simulink model "MMC_SimpleModel_20250505"  (R2024b)
settings: Solver=VariableStepAuto  StartTime=0.0  StopTime=0.5  RelTol=1e-3
values from neighbouring files (symbols this model uses):
  a = 1    [param_allsim_20250429.m]
  f0 = 50    [param_allsim_20250429.m]
  L_ac = 100e-6    (= 0.0001)    [param_allsim_20250429.m]
  L_arm = 1e-3    (= 0.001)    [param_allsim_20250429.m]
  m = 1    [param_allsim_20250429.m]
  R = 1e-6    (= 1e-06)    [param_allsim_20250429.m]
  R_ac = 1    [param_allsim_20250429.m]
  R_arm = 1e-2    (= 0.01)    [param_allsim_20250429.m]
  VDC = 800    [param_allsim_20250429.m]
undefined symbols (not defined in the file or in its folder): C_SM, L
libraries: spsSeriesRLCBranchLib x8, spsCurrentMeasurementLib x7, spsControlledVoltageSourceLib x6, spsVoltageMeasurementLib x4, spsDCVoltageSourceLib x2, spsGroundLib x1, spsThreePhaseSeriesRLCBranchLib x1, spsThreePhaseVIMeasurementLib x1, spspowerguiLib x1
settings Model: Creator=ana  LastModifiedBy=ana

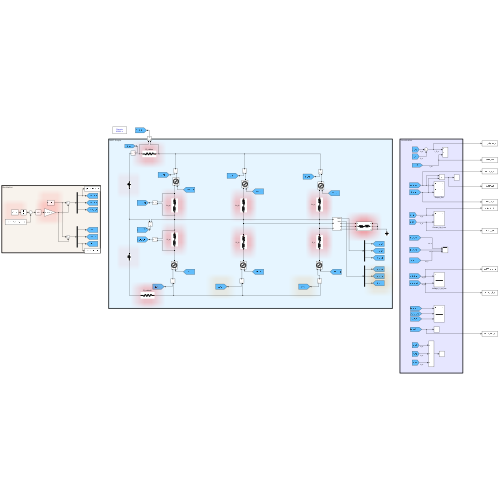
[thumbnail: Simulink's stored preview of the top-level diagram]
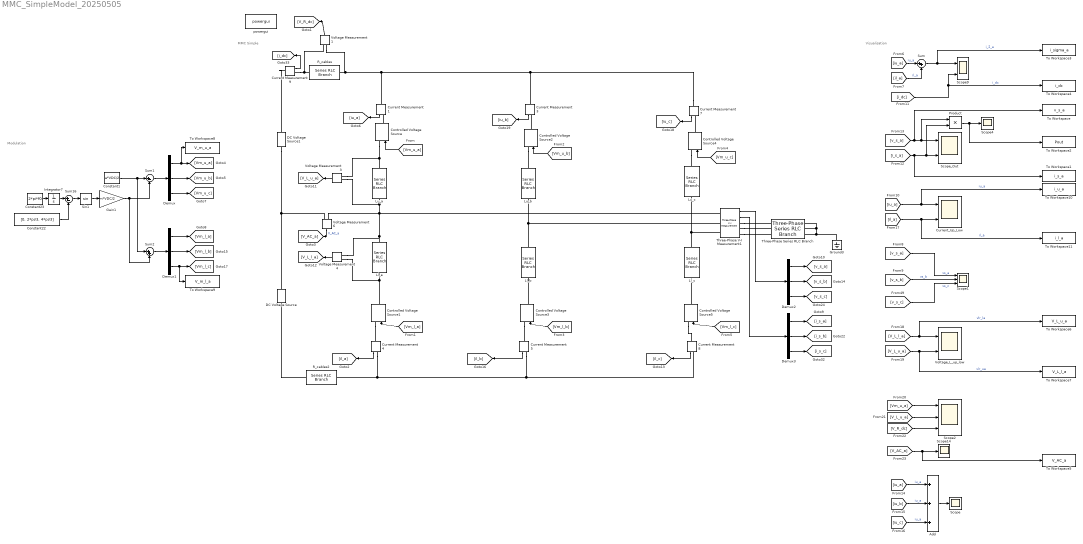
== system MMC_SimpleModel_20250505 ==
  note: Visualisation
  note: MMC Simple
  note: Modulation
  Add : Sum  Inputs=+++
  Constant1 : Constant  Value=a*VDC/2
  Constant22 : Constant  Value=[0, 2*pi/3, 4*pi/3]
  Constant23 : Constant  Value=2*pi*f0
  Controlled Voltage Source{,1..5} (6 alike) : spsControlledVoltageSourceLib/Controlled Voltage Source  Initialize=on  Source_Type=AC  Amplitude=0  Phase=0  Frequency=0  Measurements=None
  Current Measurement{1,3..5,7..9} (7 alike) : spsCurrentMeasurementLib/Current Measurement  PhasorSimulation=off  OutputType=Complex  PSBequivalent=0
  Current_Up_Low : Scope  NumInputPorts=2
  DC Voltage Source : spsDCVoltageSourceLib/DC Voltage Source  Amplitude=VDC/2  Measurements=None
  DC Voltage Source1 : spsDCVoltageSourceLib/DC Voltage Source  Amplitude=VDC/2  Measurements=None
  Demux{,1..3} (4 alike) : Demux  Outputs=3
  Gain1 : Gain  Gain=m*VDC/2
  Ground3 : spsGroundLib/Ground  LConnTagsString=a
  Integrator7 : Integrator
  Ll_a : spsSeriesRLCBranchLib/Series RLC Branch  LConnTagsString=__new0  RConnTagsString=__new0  BranchType=RL  Resistance=R_arm  Inductance=L_arm  SetiL0=off  InitialCurrent=0  Capacitance=C_SM  Setx0=off  InitialVoltage=0  Measurements=None
  Ll_b : spsSeriesRLCBranchLib/Series RLC Branch  LConnTagsString=__new0  RConnTagsString=__new0  BranchType=RL  Resistance=R_arm  Inductance=L_arm  SetiL0=off  InitialCurrent=0  Capacitance=C_SM  Setx0=off  InitialVoltage=0  Measurements=None
  Ll_c : spsSeriesRLCBranchLib/Series RLC Branch  LConnTagsString=__new0  RConnTagsString=__new0  BranchType=RL  Resistance=R_arm  Inductance=L_arm  SetiL0=off  InitialCurrent=0  Capacitance=C_SM  Setx0=off  InitialVoltage=0  Measurements=None
  Lu_a : spsSeriesRLCBranchLib/Series RLC Branch  LConnTagsString=__new0  RConnTagsString=__new0  BranchType=RL  Resistance=R_arm  Inductance=L_arm  SetiL0=on  InitialCurrent=0  Capacitance=C_SM  Setx0=off  InitialVoltage=0  Measurements=Branch voltage and current
  Lu_b : spsSeriesRLCBranchLib/Series RLC Branch  LConnTagsString=__new0  RConnTagsString=__new0  BranchType=RL  Resistance=R_arm  Inductance=L_arm  SetiL0=on  InitialCurrent=0  Capacitance=C_SM  Setx0=off  InitialVoltage=0  Measurements=Branch voltage and current
  Lu_c : spsSeriesRLCBranchLib/Series RLC Branch  LConnTagsString=__new0  RConnTagsString=__new0  BranchType=RL  Resistance=R_arm  Inductance=L_arm  SetiL0=on  InitialCurrent=0  Capacitance=C_SM  Setx0=off  InitialVoltage=0  Measurements=Branch voltage and current
  Product : Product
  R_cables : spsSeriesRLCBranchLib/Series RLC Branch  LConnTagsString=__new0  RConnTagsString=__new0  BranchType=R  Resistance=R  Inductance=L  SetiL0=on  InitialCurrent=0  Capacitance=C_SM  Setx0=off  InitialVoltage=0  Measurements=Branch voltage and current
  R_cables2 : spsSeriesRLCBranchLib/Series RLC Branch  LConnTagsString=__new0  RConnTagsString=__new0  BranchType=R  Resistance=R  Inductance=L  SetiL0=on  InitialCurrent=0  Capacitance=C_SM  Setx0=off  InitialVoltage=0  Measurements=Branch voltage and current
  Scope : Scope
  Scope1 : Scope  NumInputPorts=3
  Scope14 : Scope
  Scope2 : Scope  NumInputPorts=3
  Scope4 : Scope
  Scope9 : Scope  NumInputPorts=2
  Scope_Out : Scope  NumInputPorts=2
  Sin1 : Trigonometry
  Sum : Sum  Inputs=|++
  Sum1 : Sum  Inputs=|+-
  Sum16 : Sum  Inputs=|+-
  Sum2 : Sum  Inputs=|++
  Three-Phase Series RLC Branch : spsThreePhaseSeriesRLCBranchLib/Three-Phase Series RLC Branch  LConnTagsString=A|B|C  RConnTagsString=A|B|C  BranchType=RL  Resistance=R_ac  Inductance=L_ac  Capacitance=1e-6  Measurements=None
  Three-Phase V-I Measurement1 : spsThreePhaseVIMeasurementLib/Three-Phase V-I Measurement  VoltageMeasurement=phase-to-ground  SetLabelV=off  LabelV=Vabc  Vpu=off  VpuLL=off  CurrentMeasurement=yes  SetLabelI=off  LabelI=Iabc  Ipu=off  Pbase=100e6  Vbase=500e3  OutputType=Complex  PhasorSimulation=off  PSBequivalent=0
  To Workspace : ToWorkspace  VariableName=v_s_a  SaveFormat=Structure With Time  SampleTime=-1
  To Workspace1 : ToWorkspace  VariableName=i_s_a  SaveFormat=Structure With Time  SampleTime=-1
  To Workspace10 : ToWorkspace  VariableName=i_u_a  SaveFormat=Structure With Time  SampleTime=-1
  To Workspace11 : ToWorkspace  VariableName=i_l_a  SaveFormat=Structure With Time  SampleTime=-1
  To Workspace2 : ToWorkspace  VariableName=Pout  SaveFormat=Structure With Time  SampleTime=-1
  To Workspace3 : ToWorkspace  VariableName=i_sigma_a  SaveFormat=Structure With Time  SampleTime=-1
  To Workspace4 : ToWorkspace  VariableName=i_dc  SaveFormat=Structure With Time  SampleTime=-1
  To Workspace5 : ToWorkspace  VariableName=V_AC_a  SaveFormat=Structure With Time  SampleTime=-1
  To Workspace6 : ToWorkspace  VariableName=V_L_u_a  SaveFormat=Structure With Time  SampleTime=-1
  To Workspace7 : ToWorkspace  VariableName=V_L_l_a  SaveFormat=Structure With Time  SampleTime=-1
  To Workspace8 : ToWorkspace  VariableName=V_m_u_a  SaveFormat=Structure With Time  SampleTime=-1
  To Workspace9 : ToWorkspace  VariableName=V_m_l_a  SaveFormat=Structure With Time  SampleTime=-1
  Voltage Measurement{1,3..4,6} (4 alike) : spsVoltageMeasurementLib/Voltage Measurement  PhasorSimulation=off  OutputType=Complex  PSBequivalent=0
  Voltage_L_up_low : Scope  NumInputPorts=2
  powergui : spspowerguiLib/powergui  Priority=1  SimulationMode=Discrete  SampleTime=1e-4  frequency=60  Iterations=50  frequencyindice=0  Pbase=100e6  ErrMax=1e-4  UnitsV=kV  UnitsW=MW  buscounter=0  FunctionMessages=off  echomessages=off  EnableUseOfTLC=off  CurrentSourceSwitches=off  DisableSnubberDevices=off  DisableRonSwitches=off  DisableVfSwitches=off  DisplayEquations=off  AutomaticDiscreteSolvers=off  SolverType=Tustin/Backward Euler (TBE)  Interpol=off  ExternalGateDelay=off  methode=off  Ts=100  x0status=blocks  SPID=on  SwTol=0  HookPort=off  NonlinearTolerance=1e-4  nMaxIteration=100  ContinueOnMaxIteration=off  RestoreLinks=warning  ResistiveCurrentMeasurement=off  Frange=[0:2:500]  Ylog=off  Xlog=on  ShowGrid=off  save=off  variable=ZData  structure=0  ZoomFFT=off  StartTime=0.0  cycles=1  DisplayStyle=1  fundamental=60  FreqAxis=off  MaxFrequency=1000  frequencyindicesteady=1  RmsSteady=1  display=off
  wires:
  Sin1/1 -> Gain1/1
  Voltage Measurement3/1 -> [V_L_u_a]
  Constant22/1 -> Sum16/2
  Demux2/2 -> [v_s_b]
  [Vm_l_b] -> Controlled Voltage Source3/1
  Gain1/1 -> Sum2/2, Sum1/2
  [iu_a] -> To Workspace10/1, Current_Up_Low/1  "iu_a"
  Demux/1 -> To Workspace8/1, [Vm_u_a]
  Demux1/2 -> [Vm_l_b]
  Current Measurement5/1 -> [il_b]
  [iu_c] -> Add/3  "iu_a"
  Sum16/1 -> Sin1/1
  Demux/2 -> [Vm_u_b]
  Current Measurement4/1 -> [il_a]
  Current Measurement7/1 -> [iu_c]
  Demux2/1 -> [v_s_a]
  Sum2/1 -> Demux1/1
  Three-Phase V-I Measurement1/1 -> Demux2/1
  Demux3/3 -> [i_s_c]
  [v_s_b] -> Scope1/2  "vs_b"
  Current Measurement9/1 -> [i_dc]
  [v_s_a] -> Scope1/1  "vs_a"
  Current Measurement1/1 -> [iu_a]
  [V_L_l_a] -> To Workspace6/1, Voltage_L_up_low/1  "vlr_la"
  [Vm_u_c] -> Controlled Voltage Source4/1
  Integrator7/1 -> Sum16/1
  [il_a] -> Sum/2  "il_a"
  Sum/1 -> To Workspace3/1, Scope9/1  "i_Σ_a"
  [Vm_l_a] -> Controlled Voltage Source1/1
  Constant23/1 -> Integrator7/1
  [iu_a] -> Sum/1  "iu_a"
  [Vm_l_c] -> Controlled Voltage Source5/1
  [v_s_a] -> To Workspace/1, Product/1, Scope_Out/1
  [Vm_u_a] -> Controlled Voltage Source/1
  [iu_a] -> Add/1  "iu_a"
  [v_s_c] -> Scope1/3  "vs_c"
  Voltage Measurement4/1 -> [V_L_l_a]
  [V_L_u_a] -> To Workspace7/1, Voltage_L_up_low/2  "vlr_ua"
  Demux3/1 -> [i_s_a]
  Demux/3 -> [Vm_u_c]
  Demux2/3 -> [v_s_c]
  [iu_b] -> Add/2  "iu_a"
  Three-Phase V-I Measurement1/2 -> Demux3/1
  Current Measurement8/1 -> [il_c]
  Constant1/1 -> Sum2/1, Sum1/1
  [Vm_u_b] -> Controlled Voltage Source2/1
  Product/1 -> To Workspace2/1, Scope4/1
  Sum1/1 -> Demux/1
  [i_s_a] -> To Workspace1/1, Product/2, Scope_Out/2
  Demux1/1 -> [Vm_l_a]
  Current Measurement3/1 -> [iu_b]
  [il_a] -> To Workspace11/1, Current_Up_Low/2  "il_a"
  Add/1 -> Scope/1
  Demux3/2 -> [i_s_b]
  [i_dc] -> To Workspace4/1, Scope9/2  "i_dc"
  Demux1/3 -> To Workspace9/1, [Vm_l_c]
  [Vm_u_a] -> Scope2/1
  [V_L_u_a] -> Scope2/2
  Voltage Measurement1/1 -> [V_R_dc]
  [V_R_dc] -> Scope2/3
  Voltage Measurement6/1 -> [V_AC_a]  "V_AC_a"
  [V_AC_a] -> To Workspace5/1, Scope14/1
  connections:
  Three-Phase Series RLC Branch/RConn3 -- Three-Phase Series RLC Branch/RConn2 -- Three-Phase Series RLC Branch/RConn1 -- Ground3/LConn1
  Ll_a/RConn1 -- Voltage Measurement4/LConn2 -- Controlled Voltage Source1/RConn1
  Voltage Measurement3/LConn1 -- Controlled Voltage Source/LConn1 -- Lu_a/LConn1
  Current Measurement7/LConn1 -- Voltage Measurement1/LConn1 -- R_cables/LConn1 -- Current Measurement1/LConn1 -- Current Measurement3/LConn1
  Lu_c/RConn1 -- Ll_c/LConn1 -- Three-Phase V-I Measurement1/LConn3
  DC Voltage Source1/LConn1 -- Voltage Measurement6/LConn2 -- DC Voltage Source/RConn1
  Voltage Measurement6/LConn1 -- Voltage Measurement3/LConn2 -- Lu_a/RConn1 -- Ll_a/LConn1 -- Voltage Measurement4/LConn1 -- Three-Phase V-I Measurement1/LConn1
  Lu_b/RConn1 -- Ll_b/LConn1 -- Three-Phase V-I Measurement1/LConn2
  Current Measurement8/RConn1 -- Current Measurement4/RConn1 -- R_cables2/LConn1 -- Current Measurement5/RConn1
  Three-Phase V-I Measurement1/RConn2 -- Three-Phase Series RLC Branch/LConn2
  Controlled Voltage Source2/RConn1 -- Current Measurement3/RConn1
  Controlled Voltage Source2/LConn1 -- Lu_b/LConn1
  Controlled Voltage Source4/RConn1 -- Current Measurement7/RConn1
  Current Measurement9/LConn1 -- DC Voltage Source1/RConn1
  Controlled Voltage Source3/LConn1 -- Current Measurement5/LConn1
  Controlled Voltage Source/RConn1 -- Current Measurement1/RConn1
  DC Voltage Source/LConn1 -- R_cables2/RConn1
  Controlled Voltage Source5/LConn1 -- Current Measurement8/LConn1
  Controlled Voltage Source1/LConn1 -- Current Measurement4/LConn1
  Three-Phase V-I Measurement1/RConn1 -- Three-Phase Series RLC Branch/LConn1
  Controlled Voltage Source4/LConn1 -- Lu_c/LConn1
  Controlled Voltage Source5/RConn1 -- Ll_c/RConn1
  Controlled Voltage Source3/RConn1 -- Ll_b/RConn1
  Three-Phase V-I Measurement1/RConn3 -- Three-Phase Series RLC Branch/LConn3
  R_cables/RConn1 -- Current Measurement9/RConn1 -- Voltage Measurement1/LConn2
